simulink model "Limited_Integrator"  (R2013a)
settings: Solver=ode1  StartTime=0.0  StopTime=Inf  FixedStep=0.001  RelTol=1e-3
PostLoadFcn:
  | , if any(exist('dsrtsu_mdlpostloadfcn', 'file') == [2, 3, 6]), try dsrtsu_mdlpostloadfcn('Execute', bdroot); catch fprintf('Error in PostLoadFcn (dsrtsu_mdlpostloadfcn) for model "%s":\n %s\n', bdroot, lasterr); end, end,
libraries: simulink x1
settings Model: DSRTSU_INTERNAL_RTI_VER=430  DSRTSU_INTERNAL_RTI_TYPE=rti1401  BufferReuse=off  Creator=schiele  LastModifiedBy=schiele
settings OptimizationCC: BlockReduction=off  OptimizeBlockIOStorage=off  BufferReuse=off  ExpressionFolding=off  LocalBlockOutputs=off
settings HardwareCC: ProdIntDivRoundTo=Zero  ProdEndianess=BigEndian  ProdHWDeviceType=Generic->Custom  TargetIntDivRoundTo=Zero  TargetEndianess=BigEndian  TargetHWDeviceType=Generic->Custom
settings RTWCC: SystemTargetFile=rti1401.tlc  MakeCommand=make_rti  TemplateMakefile=rti1401.tmf  Description=dSPACE DS1401 Hardware Platform  ProcessScript=rti1401_make_rtw_hook
settings STFCustomTargetCC: ParMdlRefBuildCompliant=on  GeneratePreprocessorConditionals=Disable all  MatFileLogging=on  GRTInterface=on  SystemTargetFile=rti1401.tlc
settings GRTTargetCC: CompOptLevelCompliant=off  ConcurrentExecutionCompliant=off  CombineOutputUpdateFcns=off  GRTInterface=on

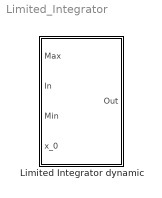
== system Limited_Integrator ==
  Limited Integrator dynamic : Subsystem

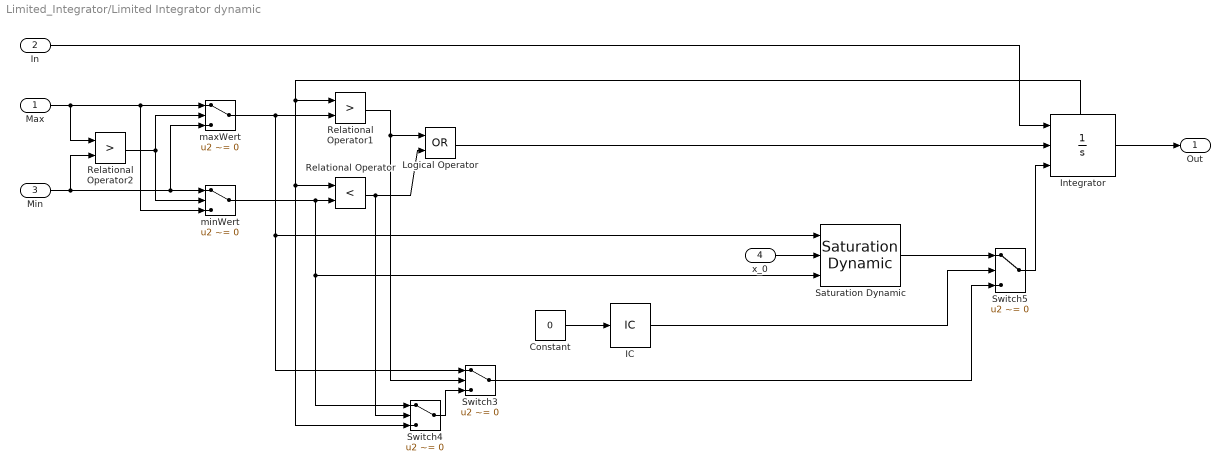
== system Limited_Integrator/Limited Integrator dynamic ==
  Max : Inport
  In : Inport  Port=2
  Min : Inport  Port=3
  x_0 : Inport  Port=4
  Constant : Constant  Value=0
  IC : InitialCondition
  Integrator : Integrator  ExternalReset=level  InitialConditionSource=external  ShowStatePort=on
  Logical Operator : Logic  Operator=OR  AllPortsSameDT=off  OutDataTypeStr=boolean
  Relational Operator : RelationalOperator  Operator=<  OutDataTypeStr=boolean
  Relational Operator1 : RelationalOperator  Operator=>  OutDataTypeStr=boolean
  Relational Operator2 : RelationalOperator  Operator=>  OutDataTypeStr=boolean
  Saturation Dynamic : simulink/Discontinuities/Saturation Dynamic  OutMin=[]  OutMax=[]  OutDataTypeStr=Inherit: Same as second input  OutDataType=fixdt(1, 16)  OutScaling=2^-10  DoSatur=off
  Switch3 : Switch  Criteria=u2 ~= 0
  Switch4 : Switch  Criteria=u2 ~= 0
  Switch5 : Switch  Criteria=u2 ~= 0
  maxWert : Switch  Criteria=u2 ~= 0
  minWert : Switch  Criteria=u2 ~= 0
  Out : Outport
  wires:
  Integrator/1 -> Out/1
  maxWert/1 -> Relational Operator1/2, Switch3/1, Saturation Dynamic/1
  minWert/1 -> Relational Operator/2, Switch4/1, Saturation Dynamic/3
  Relational Operator1/1 -> Logical Operator/1, Switch3/2
  Relational Operator/1 -> Logical Operator/2, Switch4/2
  Max/1 -> minWert/3, maxWert/1, Relational Operator2/1
  Min/1 -> minWert/1, maxWert/3, Relational Operator2/2
  Relational Operator2/1 -> maxWert/2, minWert/2
  In/1 -> Integrator/1
  Integrator/State -> Relational Operator1/1, Relational Operator/1, Switch4/3
  Switch4/1 -> Switch3/3
  Logical Operator/1 -> Integrator/2
  Switch5/1 -> Integrator/3
  x_0/1 -> Saturation Dynamic/2
  Constant/1 -> IC/1
  Saturation Dynamic/1 -> Switch5/1
  IC/1 -> Switch5/2
  Switch3/1 -> Switch5/3
